simulink model "PD_control_system"  (R2014a)
settings: Solver=ode45  StartTime=0.0  StopTime=20  RelTol=1e-3
settings Model: Creator=Huanglei  LastModifiedBy=Huanglei

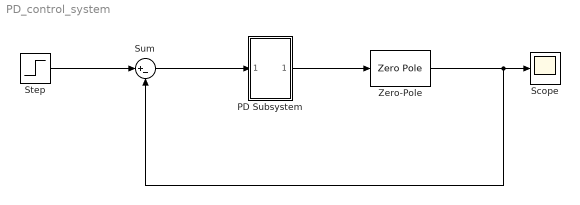
== system PD_control_system ==
  PD Subsystem : Subsystem
  Scope : Scope
      settings: TimeRange=20
  Step : Step  SampleTime=0
  Sum : Sum  Inputs=|+-
  Zero-Pole : ZeroPole  Zeros=[]  Poles=[0 -0.5]
  wires:
  Step/1 -> Sum/1
  Zero-Pole/1 -> Sum/2, Scope/1
  Sum/1 -> PD Subsystem/1(In1)
  PD Subsystem/1(Out1) -> Zero-Pole/1

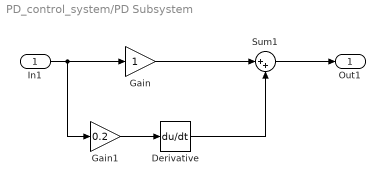
== system PD_control_system/PD Subsystem ==
  In1 : Inport
  Derivative : Derivative
  Gain : Gain
  Gain1 : Gain  Gain=0.2
  Sum1 : Sum  Inputs=|++
  Out1 : Outport
  wires:
  Gain/1 -> Sum1/1
  In1/1 -> Gain1/1, Gain/1
  Sum1/1 -> Out1/1
  Derivative/1 -> Sum1/2
  Gain1/1 -> Derivative/1
